simulink model "OPC_UA_block_converter"  (R2024b)
settings: Solver=FixedStepAuto  StartTime=0.0  StopTime=1  FixedStep=0.01  RelTol=1e-3
undefined symbols (not defined in the file or in its folder): DiscIntNeverNeededParam
libraries: simulink x3
settings Model: Creator=student  LastModifiedBy=student
settings OptimizationCC: DefaultParameterBehavior=Inlined  EnhancedBackFolding=on  PassReuseOutputArgsAs=Individual arguments  ZeroExternalMemoryAtStartup=off  ZeroInternalMemoryAtStartup=off  OptimizeBlockOrder=speed  DifferentSizesBufferReuse=on  OptimizationCustomize=off  EfficientTunableParamExpr=on
settings DebuggingCC: ParameterTunabilityLossMsg=error
settings SFSimCC: MATLABDynamicMemAlloc=off
settings RTWCC: Description=Create Visual C/C++ Solution File for Embedded Coder  SystemTargetFile=ert.tlc  TemplateMakefile=RTW.MSVCBuild
settings CodeAppCC: ForceParamTrailComments=on  IgnoreCustomStorageClasses=off  OperatorAnnotations=on  SimulinkDataObjDesc=on  SFDataObjDesc=on  InsertBlockDesc=on
settings ERTTargetCC: TargetLangStandard=C99 (ISO)  GenerateSampleERTMain=on  SupportContinuousTime=on  ERTCustomFileTemplate=example_file_process.tlc
settings ConfigComp: PLC_TargetIDE=plcopen  PLC_MultiTBSigbuilderTimeRange=off  PLC_FoldFBCallOutputVar=off  PLC_RemoveUnusedSSMethodCallArguments=off  PLC_UseCallOutputArgSyntax=off  PLC_EnableUnsignedAndDoubleTypes=off  PLC_EnableUDTSplitting=off  PLC_MaxFieldsInUDT=500  PLC_InlineEnumCastFunction=off

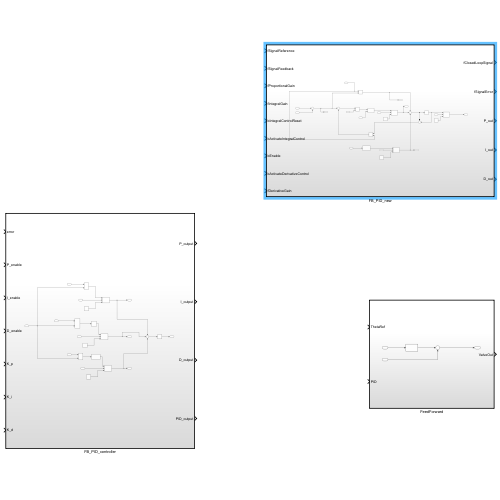
[thumbnail: Simulink's stored preview of the top-level diagram]
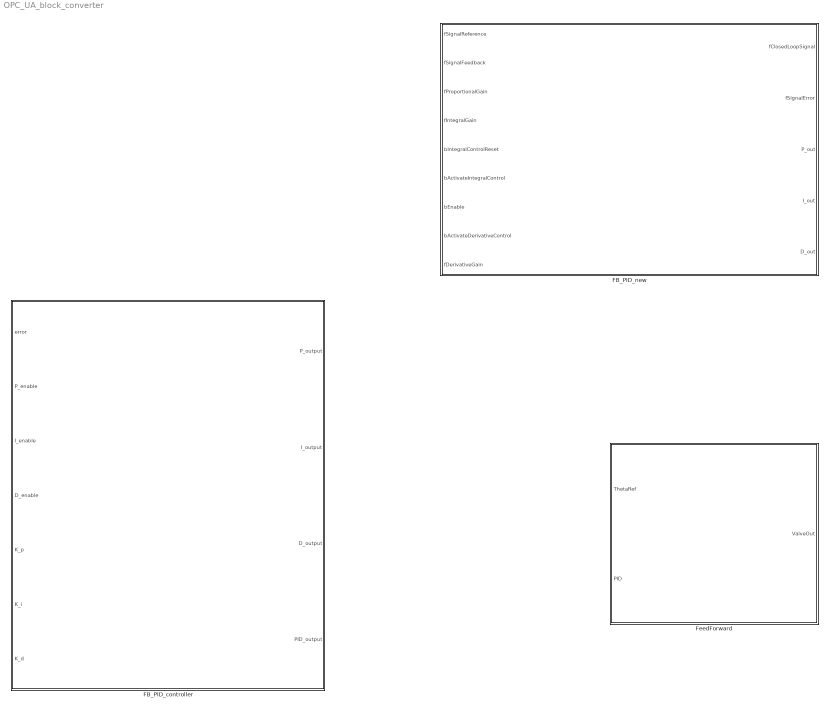
== system OPC_UA_block_converter ==
  FB_PID_controller : Subsystem  TreatAsAtomicUnit=on
  FB_PID_new : Subsystem  TreatAsAtomicUnit=on
  FeedForward : Subsystem  TreatAsAtomicUnit=on

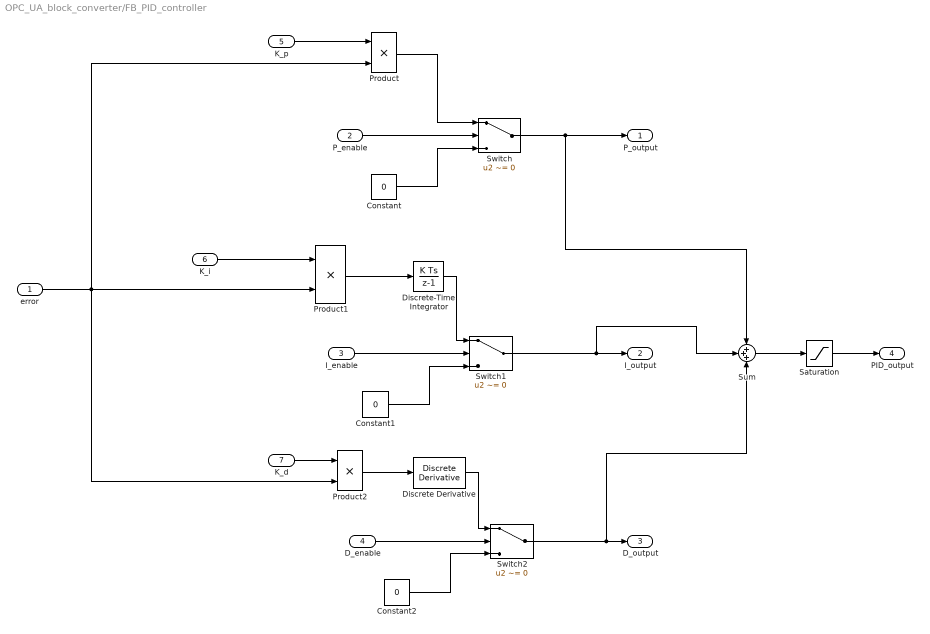
== system OPC_UA_block_converter/FB_PID_controller ==
  error : Inport
  P_enable : Inport  Port=2  OutDataTypeStr=boolean
  I_enable : Inport  Port=3  OutDataTypeStr=boolean
  D_enable : Inport  Port=4  OutDataTypeStr=boolean
  K_p : Inport  Port=5
  K_i : Inport  Port=6
  K_d : Inport  Port=7
  Constant : Constant  Value=0
  Constant1 : Constant  Value=0
  Constant2 : Constant  Value=0
  Discrete Derivative : simulink/Discrete/Discrete Derivative  gainval=1.0  ICPrevScaledInput=0.0  OutMin=[]  OutMax=[]  OutDataType=fixdt(1, 16)  OutScaling=2^-10  DoSatur=off
  Discrete-Time Integrator : DiscreteIntegrator  SampleTime=-1  ICPrevOutput=DiscIntNeverNeededParam  ICPrevScaledInput=DiscIntNeverNeededParam
  Product : Product
  Product1 : Product
  Product2 : Product
  Saturation : Saturate  UpperLimit=1  LowerLimit=-1
  Sum : Sum  Inputs=+++
  Switch : Switch  Criteria=u2 ~= 0  SaturateOnIntegerOverflow=off  InputSameDT=off
  Switch1 : Switch  Criteria=u2 ~= 0  SaturateOnIntegerOverflow=off  InputSameDT=off
  Switch2 : Switch  Criteria=u2 ~= 0  SaturateOnIntegerOverflow=off  InputSameDT=off
  P_output : Outport
  I_output : Outport  Port=2
  D_output : Outport  Port=3
  PID_output : Outport  Port=4
  wires:
  Product1/1 -> Discrete-Time Integrator/1
  error/1 -> Product2/2, Product/2, Product1/2
  Switch/1 -> Sum/1, P_output/1
  P_enable/1 -> Switch/2
  Product/1 -> Switch/1
  Constant/1 -> Switch/3
  Constant1/1 -> Switch1/3
  Discrete-Time Integrator/1 -> Switch1/1
  I_enable/1 -> Switch1/2
  Switch1/1 -> Sum/2, I_output/1
  Switch2/1 -> Sum/3, D_output/1
  D_enable/1 -> Switch2/2
  Discrete Derivative/1 -> Switch2/1
  Constant2/1 -> Switch2/3
  K_p/1 -> Product/1
  K_d/1 -> Product2/1
  Product2/1 -> Discrete Derivative/1
  K_i/1 -> Product1/1
  Sum/1 -> Saturation/1
  Saturation/1 -> PID_output/1

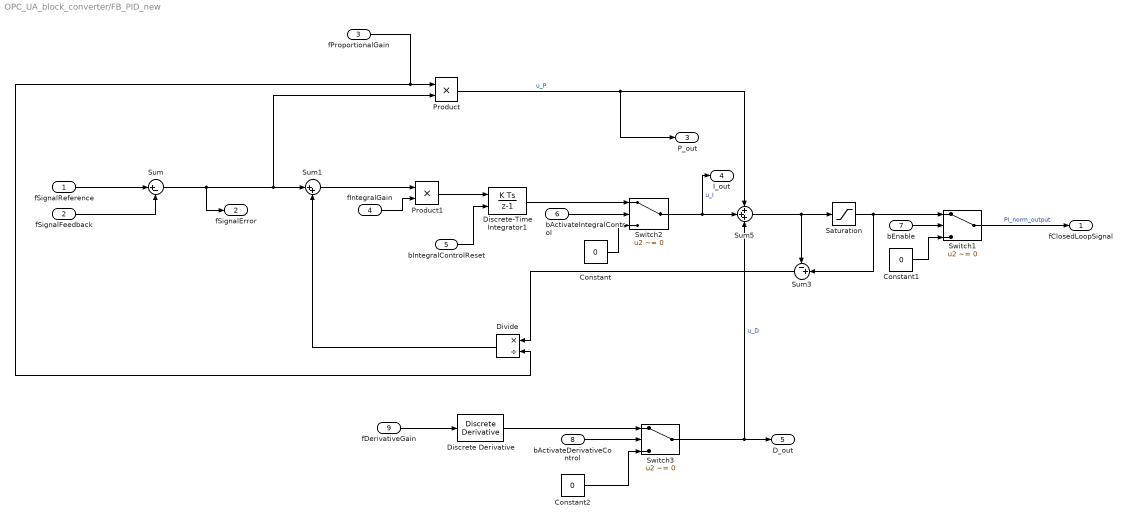
== system OPC_UA_block_converter/FB_PID_new ==
  fSignalReference : Inport
  fSignalFeedback : Inport  Port=2
  fProportionalGain : Inport  Port=3
  fIntegralGain : Inport  Port=4
  bIntegralControlReset : Inport  Port=5  OutDataTypeStr=boolean
  bActivateIntegralControl : Inport  Port=6  OutDataTypeStr=boolean
  bEnable : Inport  Port=7  OutDataTypeStr=boolean
  bActivateDerivativeControl : Inport  Port=8  OutDataTypeStr=boolean
  fDerivativeGain : Inport  Port=9
  Constant : Constant  Value=0
  Constant1 : Constant  Value=0
  Constant2 : Constant  Value=0
  Discrete Derivative : simulink/Discrete/Discrete Derivative  gainval=1.0  ICPrevScaledInput=0.0  OutMin=[]  OutMax=[]  OutDataType=fixdt(1, 16)  OutScaling=2^-10  DoSatur=off
  Discrete-Time Integrator1 : DiscreteIntegrator  ExternalReset=sampled level  SampleTime=-1  LimitOutput=on  UpperSaturationLimit=1  LowerSaturationLimit=-1  ICPrevOutput=DiscIntNeverNeededParam  ICPrevScaledInput=DiscIntNeverNeededParam
  Divide : Product  Inputs=*/
  Product : Product
  Product1 : Product
  Saturation : Saturate  UpperLimit=1  LowerLimit=-1
  Sum : Sum  Inputs=|+-
  Sum1 : Sum  Inputs=|++
  Sum3 : Sum  Inputs=-+|
  Sum5 : Sum  Inputs=+++
  Switch1 : Switch  Criteria=u2 ~= 0  SaturateOnIntegerOverflow=off  InputSameDT=off
  Switch2 : Switch  Criteria=u2 ~= 0  SaturateOnIntegerOverflow=off  InputSameDT=off
  Switch3 : Switch  Criteria=u2 ~= 0  SaturateOnIntegerOverflow=off  InputSameDT=off
  fClosedLoopSignal : Outport
  fSignalError : Outport  Port=2
  P_out : Outport  Port=3
  I_out : Outport  Port=4
  D_out : Outport  Port=5
  wires:
  fSignalReference/1 -> Sum/1
  fSignalFeedback/1 -> Sum/2
  Sum/1 -> fSignalError/1, Product/2, Sum1/1
  fProportionalGain/1 -> Product/1, Divide/2
  Sum1/1 -> Product1/1
  fIntegralGain/1 -> Product1/2
  Product1/1 -> Discrete-Time Integrator1/1
  bIntegralControlReset/1 -> Discrete-Time Integrator1/2
  Discrete-Time Integrator1/1 -> Switch2/1
  bActivateIntegralControl/1 -> Switch2/2
  Constant/1 -> Switch2/3
  Product/1 -> P_out/1, Sum5/1  "u_P"
  Switch2/1 -> I_out/1, Sum5/2  "u_I"
  Sum5/1 -> Sum3/1, Saturation/1
  Saturation/1 -> Switch1/1, Sum3/2
  Sum3/1 -> Divide/1
  Divide/1 -> Sum1/2
  bEnable/1 -> Switch1/2
  Constant1/1 -> Switch1/3
  Switch1/1 -> fClosedLoopSignal/1  "PI_norm_output"
  Constant2/1 -> Switch3/3
  Discrete Derivative/1 -> Switch3/1
  bActivateDerivativeControl/1 -> Switch3/2
  fDerivativeGain/1 -> Discrete Derivative/1
  Switch3/1 -> D_out/1, Sum5/3  "u_D"

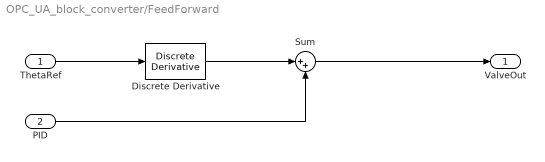
== system OPC_UA_block_converter/FeedForward ==
  ThetaRef : Inport
  PID : Inport  Port=2
  Discrete Derivative : simulink/Discrete/Discrete Derivative  gainval=1.0  ICPrevScaledInput=0.0  OutMin=[]  OutMax=[]  OutDataType=fixdt(1, 16)  OutScaling=2^-10  DoSatur=off
  Sum : Sum  Inputs=|++
  ValveOut : Outport
  wires:
  ThetaRef/1 -> Discrete Derivative/1
  Sum/1 -> ValveOut/1
  Discrete Derivative/1 -> Sum/1
  PID/1 -> Sum/2
